simulink model "T50_DD"  (R2016b)
settings: configuration reference "CodeGenConfigSet" (kept outside this file)
values from neighbouring files (symbols this model uses):
  T50_tiDebHiLo_C = Calibration.Parameter    [init_T50_DD.m]    (also in init_T50_DD_SIL.m = Simulink.Parameter)
  T50_tiDebLoHi_C = Calibration.Parameter    [init_T50_DD.m]    (also in init_T50_DD_SIL.m = Simulink.Parameter)
  T50_uThreshold_C = Calibration.Parameter    [init_T50_DD.m]    (also in init_T50_DD_SIL.m = Simulink.Parameter)
undefined symbols (not defined in the file or in its folder): T50_DD_DT
libraries: CXLib x1
settings Model: Creator=xuxingpei  LastModifiedBy=guanxiaoxing
settings ConfigSetRef: SourceLocation=Base Workspace

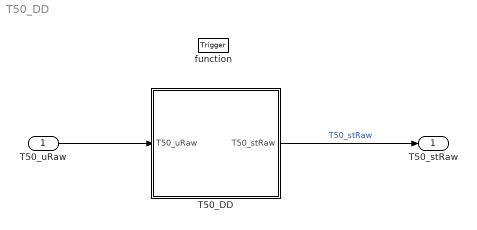
== system T50_DD ==
  T50_uRaw : Inport  Tag=mv  Description=Raw ADC value of downstream engine coolant temperature sensor signal  OutMin=0  OutMax=5000  OutDataTypeStr=Ad_mv
  function : TriggerPort  TriggerType=function-call  VariantControl=Variant
  T50_DD : Subsystem
  T50_stRaw : Outport  Description=Terminal 50 status after debouncing  OutDataTypeStr=Enum: Switch_conv
  wires:
  T50_uRaw/1 -> T50_DD/1(T50_uRaw)
  T50_DD/1(T50_stRaw) -> T50_stRaw/1  "T50_stRaw"

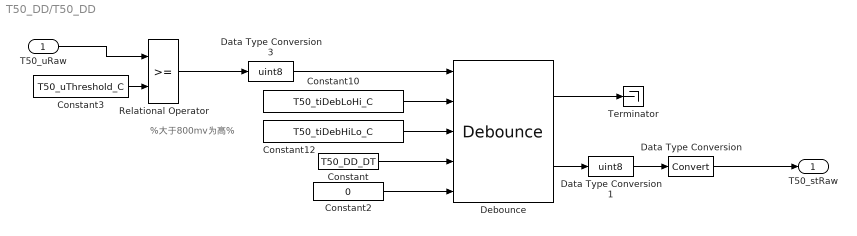
== system T50_DD/T50_DD ==
  note: %大于800mv为高%
  T50_uRaw : Inport  Tag=mv  Description=Raw ADC value of downstream engine coolant temperature sensor signal  OutMin=0  OutMax=5000  OutDataTypeStr=Ad_mv
  Constant : Constant  Value=T50_DD_DT
  Constant10 : Constant  Value=T50_tiDebLoHi_C
  Constant12 : Constant  Value=T50_tiDebHiLo_C
  Constant2 : Constant  Value=0  OutDataTypeStr=Inherit: Inherit via back propagation
  Constant3 : Constant  Value=T50_uThreshold_C
  Data Type Conversion : DataTypeConversion
  Data Type Conversion1 : DataTypeConversion  OutDataTypeStr=uint8
  Data Type Conversion3 : DataTypeConversion  OutDataTypeStr=uint8
  Debounce : CXLib/Debounce
  Relational Operator : RelationalOperator  OutDataTypeStr=boolean  RndMeth=Nearest  InputSameDT=on
  Terminator : Terminator
  T50_stRaw : Outport  Description=Terminal 50 status after debouncing  OutDataTypeStr=Enum: Switch_conv
  wires:
  Constant/1 -> Debounce/4
  T50_uRaw/1 -> Relational Operator/1
  Debounce/2 -> Data Type Conversion1/1
  Relational Operator/1 -> Data Type Conversion3/1
  Constant12/1 -> Debounce/3
  Data Type Conversion/1 -> T50_stRaw/1
  Constant2/1 -> Debounce/5
  Data Type Conversion1/1 -> Data Type Conversion/1
  Constant3/1 -> Relational Operator/2
  Debounce/1 -> Terminator/1
  Constant10/1 -> Debounce/2
  Data Type Conversion3/1 -> Debounce/1
